simulink subsystem "Lift_Cruise_Reference_Inputs"  (R2022b)
settings: Solver=VariableStepAuto  StartTime=0.0  StopTime=10.0  RelTol=1e-3
libraries: DoubletsLib x3
settings Model: Creator=tbritton  LastModifiedBy=macheson
settings SolverCC: AlgebraicLoopSolver=TrustRegion
settings DebuggingCC: UnconnectedInputMsg=warning  UnconnectedOutputMsg=warning  UnconnectedLineMsg=warning  SFMachineParentedDataDiag=warning
settings ModelReferenceCC: EnableRefExpFcnMdlSchedulingChecks=on
settings RTWCC: DLArmComputeVersion=19.05

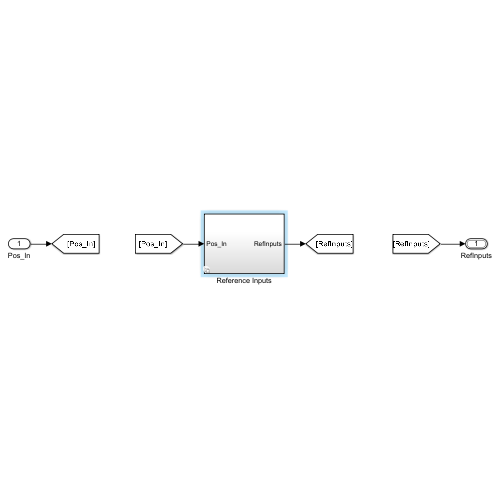
[thumbnail: Simulink's stored preview of the top-level diagram]
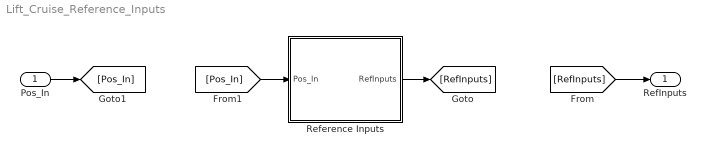
== system Lift_Cruise_Reference_Inputs ==
  Pos_In : Inport
  Reference Inputs : Subsystem  Variant=on
  RefInputs : Outport  OutDataTypeStr=Bus: BUS_REF_INPUT  VectorParamsAs1DForOutWhenUnconnected=off
  wires:
  [RefInputs] -> RefInputs/1
  Reference Inputs/1(RefInputs) -> [RefInputs]
  [Pos_In] -> Reference Inputs/1(Pos_In)
  Pos_In/1 -> [Pos_In]

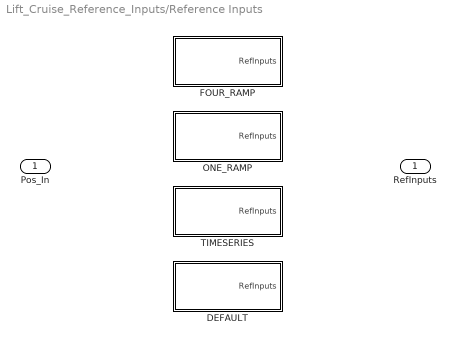
== system Lift_Cruise_Reference_Inputs/Reference Inputs ==
  Pos_In : Inport
  DEFAULT : Subsystem  VariantControl=GVS_REFINPUT_TYPE_DEFAULT
  FOUR_RAMP : Subsystem  VariantControl=GVS_REFINPUT_TYPE_4RAMP
  ONE_RAMP : Subsystem  VariantControl=GVS_REFINPUT_TYPE_1RAMP
  TIMESERIES : Subsystem  VariantControl=GVS_REFINPUT_TYPE_TIMESERIES
  RefInputs : Outport  OutDataTypeStr=Bus: BUS_REF_INPUT  VectorParamsAs1DForOutWhenUnconnected=off

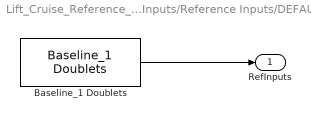
== system Lift_Cruise_Reference_Inputs/Reference Inputs/DEFAULT ==
  Baseline_1 Doublets : DoubletsLib/Baseline_1 Doublets  SystemSampleTime=-1  VariantActivationTime=update diagram  Latency=0  AutoFrameSizeCalculation=off
  RefInputs : Outport
  wires:
  Baseline_1 Doublets/1 -> RefInputs/1

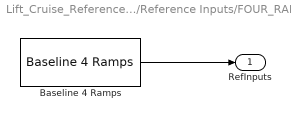
== system Lift_Cruise_Reference_Inputs/Reference Inputs/FOUR_RAMP ==
  Baseline 4 Ramps : DoubletsLib/Baseline 4 Ramps  SystemSampleTime=-1  VariantActivationTime=update diagram  Latency=0  AutoFrameSizeCalculation=off
  RefInputs : Outport
  wires:
  Baseline 4 Ramps/1 -> RefInputs/1

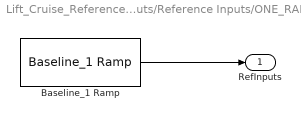
== system Lift_Cruise_Reference_Inputs/Reference Inputs/ONE_RAMP ==
  Baseline_1 Ramp : DoubletsLib/Baseline_1 Ramp  SystemSampleTime=-1  VariantActivationTime=update diagram  Latency=0  AutoFrameSizeCalculation=off
  RefInputs : Outport
  wires:
  Baseline_1 Ramp/1 -> RefInputs/1

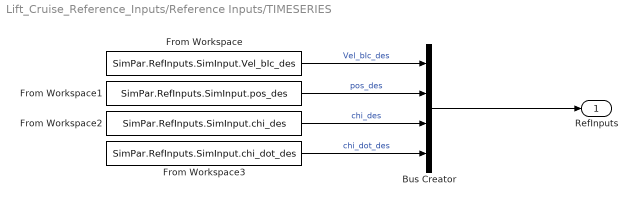
== system Lift_Cruise_Reference_Inputs/Reference Inputs/TIMESERIES ==
  Bus Creator : BusCreator  Inputs=4
  From Workspace : FromWorkspace  VariableName=SimPar.RefInputs.SimInput.Vel_bIc_des  OutputAfterFinalValue=Holding final value
  From Workspace1 : FromWorkspace  VariableName=SimPar.RefInputs.SimInput.pos_des  OutputAfterFinalValue=Holding final value
  From Workspace2 : FromWorkspace  VariableName=SimPar.RefInputs.SimInput.chi_des  OutputAfterFinalValue=Holding final value
  From Workspace3 : FromWorkspace  VariableName=SimPar.RefInputs.SimInput.chi_dot_des  OutputAfterFinalValue=Holding final value
  RefInputs : Outport
  wires:
  Bus Creator/1 -> RefInputs/1
  From Workspace3/1 -> Bus Creator/4  "chi_dot_des"
  From Workspace2/1 -> Bus Creator/3  "chi_des"
  From Workspace1/1 -> Bus Creator/2  "pos_des"
  From Workspace/1 -> Bus Creator/1  "Vel_bIc_des"
